simulink model "TC_model"  (R2013a)
settings: Solver=ode45  StartTime=0.0  StopTime=10.0  RelTol=1e-3
undefined symbols (not defined in the file): ctrl_sat, DiscIntNeverNeededParam
libraries: powerlib x7
settings Model: CovModelRefEnable=off  Creator=Copy864  LastModifiedBy=Copy864
settings DataIOCC: LimitDataPoints=off  SaveFormat=StructureWithTime
settings DebuggingCC: UnderspecifiedInitializationDetection=Simplified  MergeDetectMultiDrivingBlocksExec=error  SolverPrmCheckMsg=none  FrameProcessingCompatibilityMsg=error  StateNameClashWarn=none
settings HardwareCC: ProdBitPerPointer=64  ProdLargestAtomicFloat=Float  ProdIntDivRoundTo=Zero  ProdEndianess=LittleEndian  ProdHWDeviceType=Specified
settings ModelReferenceCC: PropagateSignalLabelsOutOfModel=on
settings GRTTargetCC: CodeReplacementLibrary=C89/C90 (ANSI)
settings ConfigurationSet: Description=Simscape Multibody

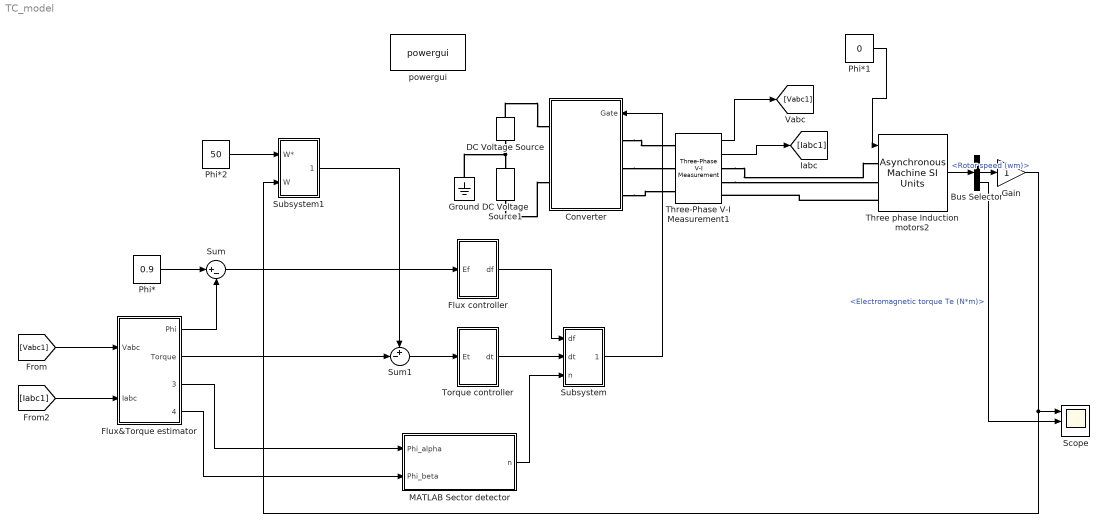
== system TC_model ==
  Bus Selector : BusSelector  OutputSignals=Stator measurements.Stator current is_a (A),Mechanical.Rotor speed (wm),Mechanical.Electromagnetic torque Te (N*m)
  Converter : Subsystem
  DC Voltage Source : powerlib/Electrical Sources/DC Voltage Source  Amplitude=250  Measurements=None
  DC Voltage Source1 : powerlib/Electrical Sources/DC Voltage Source  Amplitude=250  Measurements=None
  Flux controller : Subsystem
  Flux&Torque estimator : Subsystem
  Gain : Gain
  Ground : powerlib/Elements/Ground  LConnTagsString=a
  MATLAB Sector detector : MATLAB Function  TreatAsAtomicUnit=on
      settings: PermitHierarchicalResolution=ParametersOnly
  Phi* : Constant  Value=0.9
  Phi*1 : Constant  Value=0
  Phi*2 : Constant  Value=50
  Scope : Scope  NumInputPorts=3
      settings: TimeRange=auto  MaxDataPoints=5000  SaveName=ScopeData  YMin=-16.0259~-157.28143~-1.00000  YMax=144.23311~146.13243~1.00000  SampleTime=-1
  Subsystem : Subsystem
  Subsystem1 : Subsystem
  Sum : Sum  Inputs=|+-
  Sum1 : Sum  Inputs=+-|
  Three phase Induction motors2 : powerlib/Machines/Asynchronous Machine SI Units  RotorType=Squirrel-cage  PresetModel=No  MechanicalLoad=Torque Tm  ShowDetailedParameters=on  ReferenceFrame=Rotor  Units=SI  MeasurementBus=off  NominalParameters=[500000 460 60]  Stator=[0.6837 0.004152]  Rotor=[0.451 0.004152]  Cage1=[0.4155 0.002066]  Cage2=[0.4168 0.0003495]  Lm=0.1486  Mechanical=[0.05 0.02791 1]  PolePairs=2  InitialConditions=[1 0 0 0 0 0 0 0]  SimulateSaturation=off  Saturation=[14.03593122, 27.81365428, 53.79336849, 72.68890987, 97.98006896, 148.6815601, 215.7428561, 302.9841135, 428.7778367 ; 230, 322, 414, 460, 506, 552, 598, 644, 690]  LoadFlowParameters=1492000  TsPowergui=0  TsBlock=2*10^-6  IterativeModel=Trapezoidal non iterative  IterativeDiscreteModel=Trapezoidal iterative (alg. loop)  Pmec=1.492e+006
  Three-Phase V-I Measurement1 : powerlib/Measurements/Three-Phase V-I Measurement  VoltageMeasurement=phase-to-ground  SetLabelV=off  LabelV=Vabc  Vpu=off  VpuLL=off  CurrentMeasurement=yes  SetLabelI=off  LabelI=Iabc  Ipu=off  Pbase=100e6  Vbase=500e3  OutputType=Complex  PhasorSimulation=off  PSBequivalent=0
  "Torque controller " : Subsystem
  powergui : powerlib/powergui  Priority=1  SimulationMode=Discrete  SolverType=Backward Euler  SampleTime=2e-6  frequency=60  SPID=on  DisableSnubberDevices=off  DisableRonSwitches=off  DisableVfSwitches=off  SwTol=0  DisplayEquations=off  Interpol=off  ExternalGateDelay=off  methode=off  Ts=100  FunctionMessages=off  echomessages=off  HookPort=off  EnableUseOfTLC=off  x0status=blocks  frequencyindice=0  Pbase=100e6  ErrMax=1e-4  Iterations=50  UnitsV=kV  UnitsW=MW  buscounter=0  RestoreLinks=warning  ResistiveCurrentMeasurement=off  Frange=[0:2:500]  Ylog=off  Xlog=on  ShowGrid=off  save=off  variable=ZData  structure=0  ZoomFFT=off  StartTime=0.0  cycles=1  DisplayStyle=1  fundamental=60  FreqAxis=off  MaxFrequency=1000  frequencyindicesteady=1  RmsSteady=1  display=off
  wires:
  Three-Phase V-I Measurement1/2 -> [Iabc1]
  [Vabc1] -> Flux&Torque estimator/1(Vabc)
  [Iabc1] -> Flux&Torque estimator/2(Iabc)
  Flux&Torque estimator/3(Phi_alpha) -> MATLAB Sector detector/1(Phi_alpha)
  Flux&Torque estimator/4(Phi_beta) -> MATLAB Sector detector/2(Phi_beta)
  Flux&Torque estimator/2(Torque) -> Sum1/2
  Flux&Torque estimator/1(Phi) -> Sum/2
  Phi*/1 -> Sum/1
  Sum/1 -> Flux controller/1(Ef)
  Sum1/1 -> "Torque controller "/1(Et)
  Flux controller/1(df) -> Subsystem/1(df)
  "Torque controller "/1(dt) -> Subsystem/2(dt)
  MATLAB Sector detector/1(n) -> Subsystem/3(n)
  Subsystem/1(Gate) -> Converter/1("Gate ")
  Three phase Induction motors2/1 -> Bus Selector/1
  Bus Selector/2 -> Gain/1  "<Rotor speed (wm)>"
  Phi*2/1 -> Subsystem1/1(W*)
  Gain/1 -> Subsystem1/2(W), Scope/1
  Bus Selector/3 -> Scope/2  "<Electromagnetic torque Te (N*m)>"
  Three-Phase V-I Measurement1/1 -> [Vabc1]
  Phi*1/1 -> Three phase Induction motors2/1
  Subsystem1/1(Te*) -> Sum1/1
  connections:
  Three phase Induction motors2/LConn3 -- Three-Phase V-I Measurement1/RConn3
  Converter/LConn2 -- Three-Phase V-I Measurement1/LConn2
  Converter/LConn1 -- Three-Phase V-I Measurement1/LConn1
  Three-Phase V-I Measurement1/RConn1 -- Three phase Induction motors2/LConn1
  Converter/LConn3 -- Three-Phase V-I Measurement1/LConn3
  Three-Phase V-I Measurement1/RConn2 -- Three phase Induction motors2/LConn2
  DC Voltage Source/RConn1 -- Converter/RConn1
  DC Voltage Source/LConn1 -- Ground/LConn1 -- DC Voltage Source1/RConn1
  DC Voltage Source1/LConn1 -- Converter/RConn2

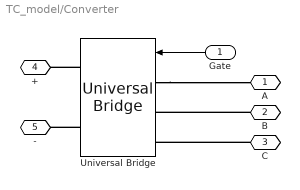
== system TC_model/Converter ==
  "Gate " : Inport
  Universal Bridge : powerlib/Power Electronics/Universal Bridge  Arms=3  SnubberResistance=1e5  SnubberCapacitance=inf  Device=IGBT / Diodes  Ron=1e-3  Lon=0  ForwardVoltages="[  0  0  ]"  ForwardVoltage=0  GTOparameters=[ 10e-6 , 20e-6 ]  IGBTparameters=[ 1e-6 , 2e-6 ]  Measurements=None  Measurements_2=None  converterType=Rectifier
  A : PMIOPort  Port=1  Side=Left
  B : PMIOPort  Port=2  Side=Left
  C : PMIOPort  Port=3  Side=Left
  + : PMIOPort  Port=4  Side=Right
  - : PMIOPort  Port=5  Side=Right
  wires:
  "Gate "/1 -> Universal Bridge/1
  connections:
  C/RConn1 -- Universal Bridge/LConn3
  Universal Bridge/RConn1 -- +/RConn1
  Universal Bridge/LConn1 -- A/RConn1
  Universal Bridge/RConn2 -- -/RConn1
  B/RConn1 -- Universal Bridge/LConn2

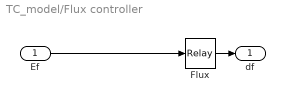
== system TC_model/Flux controller ==
  Ef : Inport
  Flux : Relay  OnSwitchValue=0.005  OffSwitchValue=-0.005
  df : Outport
  wires:
  Ef/1 -> Flux/1
  Flux/1 -> df/1

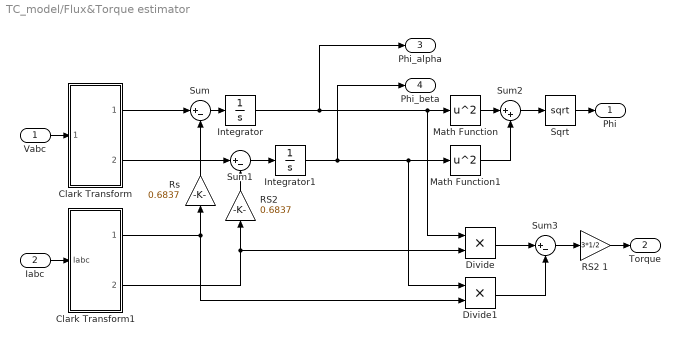
== system TC_model/Flux&Torque estimator ==
  Vabc : Inport
  Iabc : Inport  Port=2
  Clark Transform : Subsystem
  Clark Transform1 : Subsystem
  Divide : Product  Inputs=**
  Divide1 : Product  Inputs=**
  Integrator : Integrator
  Integrator1 : Integrator
  Math Function : Math  Operator=square  SaturateOnIntegerOverflow=on
  Math Function1 : Math  Operator=square  SaturateOnIntegerOverflow=on
  "RS2 " : Gain  Gain=0.6837
  RS2 1 : Gain  Gain=3*1/2
  Rs : Gain  Gain=0.6837
  Sqrt : Sqrt  SaturateOnIntegerOverflow=on
  Sum : Sum  Inputs=|+-
  Sum1 : Sum  Inputs=|+-
  Sum2 : Sum  Inputs=|++
  Sum3 : Sum  Inputs=|+-
  Phi : Outport
  Torque : Outport  Port=2
  Phi_alpha : Outport  Port=3
  Phi_beta : Outport  Port=4
  wires:
  Math Function1/1 -> Sum2/2
  Sum2/1 -> Sqrt/1
  Integrator/1 -> Phi_alpha/1, Divide/1, Math Function/1
  RS2 1/1 -> Torque/1
  Clark Transform1/2("Ibeta ") -> "RS2 "/1, Divide/2
  Rs/1 -> Sum/2
  "RS2 "/1 -> Sum1/2
  Clark Transform1/1(Ialpha) -> Divide1/2, Rs/1
  Divide/1 -> Sum3/1
  Integrator1/1 -> Phi_beta/1, Divide1/1, Math Function1/1
  Sum1/1 -> Integrator1/1
  Math Function/1 -> Sum2/1
  Clark Transform/1(Valpha) -> Sum/1
  Clark Transform/2("Vbeta ") -> Sum1/1
  Divide1/1 -> Sum3/2
  Sum/1 -> Integrator/1
  Sum3/1 -> RS2 1/1
  Vabc/1 -> Clark Transform/1(Vabc)
  Iabc/1 -> Clark Transform1/1(Iabc)
  Sqrt/1 -> Phi/1

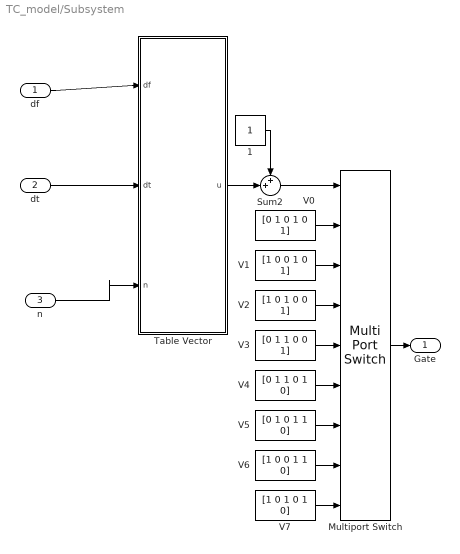
== system TC_model/Subsystem ==
  df : Inport
  dt : Inport  Port=2
  n : Inport  Port=3
  1 : Constant
  Multiport Switch : MultiPortSwitch  Inputs=8
  Sum2 : Sum  Inputs=++|
  Table Vector : MATLAB Function  TreatAsAtomicUnit=on
      settings: PermitHierarchicalResolution=ParametersOnly
  V0 : Constant  Value=[0 1 0 1 0 1]
  V1 : Constant  Value=[1 0 0 1 0 1]
  V2 : Constant  Value=[1 0 1 0 0 1]
  "V3 " : Constant  Value=[0 1 1 0 0 1]
  V4 : Constant  Value=[0 1 1 0 1 0]
  V5 : Constant  Value=[0 1 0 1 1 0]
  V6 : Constant  Value=[1 0 0 1 1 0]
  V7 : Constant  Value=[1 0 1 0 1 0]
  Gate : Outport
  wires:
  "V3 "/1 -> Multiport Switch/5
  V7/1 -> Multiport Switch/9
  V5/1 -> Multiport Switch/7
  1/1 -> Sum2/1
  V2/1 -> Multiport Switch/4
  V1/1 -> Multiport Switch/3
  dt/1 -> Table Vector/2(dt)
  V4/1 -> Multiport Switch/6
  V0/1 -> Multiport Switch/2
  Table Vector/1(u) -> Sum2/2
  Sum2/1 -> Multiport Switch/1
  V6/1 -> Multiport Switch/8
  n/1 -> Table Vector/3(n)
  Multiport Switch/1 -> Gate/1
  df/1 -> Table Vector/1(df)

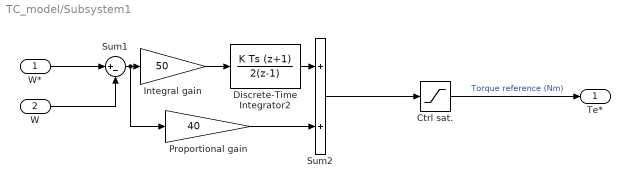
== system TC_model/Subsystem1 ==
  W* : Inport
  W : Inport  Port=2
  Ctrl sat. : Saturate  UpperLimit=1e6  LowerLimit=-2000
  Discrete-Time Integrator2 : DiscreteIntegrator  IntegratorMethod=Integration: Trapezoidal  SampleTime=-1  UpperSaturationLimit=ctrl_sat(2)  LowerSaturationLimit=ctrl_sat(1)  ICPrevOutput=DiscIntNeverNeededParam  ICPrevScaledInput=DiscIntNeverNeededParam
  Integral gain : Gain  Gain=50  SaturateOnIntegerOverflow=on  OutDataTypeStr=Inherit: Same as input  ParamDataTypeStr=Inherit: Same as input
  Proportional gain : Gain  Gain=40  SaturateOnIntegerOverflow=on  OutDataTypeStr=Inherit: Same as input  ParamDataTypeStr=Inherit: Same as input
  Sum1 : Sum  Inputs=|+-  SaturateOnIntegerOverflow=on  InputSameDT=on  OutDataTypeStr=Inherit: Same as first input
  Sum2 : Sum  SaturateOnIntegerOverflow=on  InputSameDT=on  OutDataTypeStr=Inherit: Same as first input
  Te* : Outport
  wires:
  Sum2/1 -> Ctrl sat./1
  Integral gain/1 -> Discrete-Time Integrator2/1
  Discrete-Time Integrator2/1 -> Sum2/1
  Sum1/1 -> Integral gain/1, Proportional gain/1
  Proportional gain/1 -> Sum2/2
  W*/1 -> Sum1/1
  W/1 -> Sum1/2
  Ctrl sat./1 -> Te*/1  "Torque reference (Nm)"

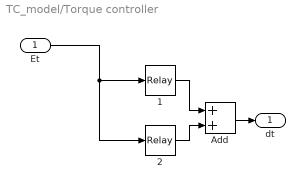
== system TC_model/Torque controller  ==
  Et : Inport
  "1 " : Relay  OnSwitchValue=1  OffSwitchValue=0
  2 : Relay  OnSwitchValue=0  OffSwitchValue=-1  OnOutputValue=0  OffOutputValue=-1
  Add : Sum
  dt : Outport
  wires:
  Et/1 -> "1 "/1, 2/1
  Add/1 -> dt/1
  "1 "/1 -> Add/1
  2/1 -> Add/2

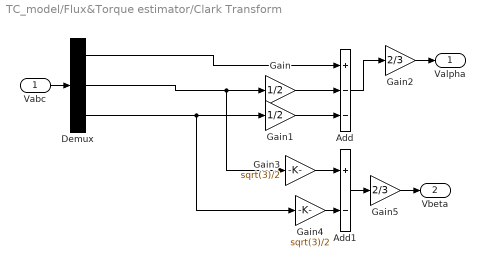
== system TC_model/Flux&Torque estimator/Clark Transform ==
  Vabc : Inport
  Add : Sum  Inputs=+--
  Add1 : Sum  Inputs=+-
  Demux : Demux  Outputs=3
  Gain : Gain  Gain=1/2
  Gain1 : Gain  Gain=1/2
  Gain2 : Gain  Gain=2/3
  Gain3 : Gain  Gain=sqrt(3)/2
  Gain4 : Gain  Gain=sqrt(3)/2
  Gain5 : Gain  Gain=2/3
  Valpha : Outport
  "Vbeta " : Outport  Port=2
  wires:
  Demux/3 -> Gain4/1, Gain1/1
  Gain1/1 -> Add/3
  Gain4/1 -> Add1/2
  Demux/1 -> Add/1
  Demux/2 -> Gain3/1, Gain/1
  Gain3/1 -> Add1/1
  Add/1 -> Gain2/1
  Gain/1 -> Add/2
  Add1/1 -> Gain5/1
  Vabc/1 -> Demux/1
  Gain2/1 -> Valpha/1
  Gain5/1 -> "Vbeta "/1

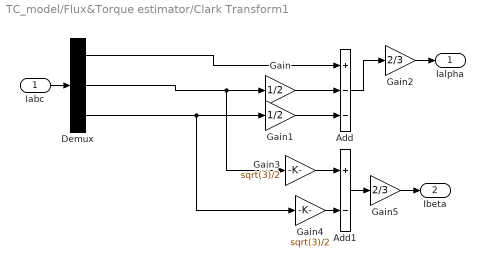
== system TC_model/Flux&Torque estimator/Clark Transform1 ==
  Iabc : Inport
  Add : Sum  Inputs=+--
  Add1 : Sum  Inputs=+-
  Demux : Demux  Outputs=3
  Gain : Gain  Gain=1/2
  Gain1 : Gain  Gain=1/2
  Gain2 : Gain  Gain=2/3
  Gain3 : Gain  Gain=sqrt(3)/2
  Gain4 : Gain  Gain=sqrt(3)/2
  Gain5 : Gain  Gain=2/3
  Ialpha : Outport
  "Ibeta " : Outport  Port=2
  wires:
  Gain5/1 -> "Ibeta "/1
  Gain2/1 -> Ialpha/1
  Iabc/1 -> Demux/1
  Add1/1 -> Gain5/1
  Gain/1 -> Add/2
  Add/1 -> Gain2/1
  Gain3/1 -> Add1/1
  Demux/2 -> Gain/1, Gain3/1
  Demux/1 -> Add/1
  Gain4/1 -> Add1/2
  Gain1/1 -> Add/3
  Demux/3 -> Gain1/1, Gain4/1

== matlab function TC_model/Subsystem/Table Vector ==
  data: df input; u output; dt input; n input
function u = fcn(df, dt , n)
u = 0;
if (df == 1) & (dt == 1) & (n == 1)
    u =2;   
end

if (df == 1) & (dt == 0) & (n == 1)
    u =7;   
end

if (df == 1) & (dt == -1) & (n == 1)
    u =6;   
end
%%%%%%%%%%%%%%%%%%%%%%%%%%%%%%%
if (df == 1) & (dt == 1) & (n == 2)
    u =3;   
end
if (df == 1) & (dt == 0) & (n == 2)
    u =0;   
end
if (df == 1) & (dt == -1) & (n == 2)
    u =1;   
end
%%%%%%%%%%%%%%%%%%%%%%%%%%%%%
if (df == 1) & (dt == 1) & (n == 3)
    u =4;   
end
if (df == 1) & (dt == 0) & (n == 3)
    u =7;   
end
if (df == 1) & (dt == -1) & (n == 3)
    u =2;   
end
%%%%%%%%%%%%%%%%%%%%%%%%%%%%%
if (df == 1) & (dt == 1) & (n == 4)
    u =5;   
end
if (df == 1) & (dt == 0) & (n == 4)
    u =0;   
end
if (df == 1) & (dt == -1) & (n == 4)
    u =3;   
end
%%%%%%%%%%%%%%%%%%%%%%%%%%%%%
if (df == 1) & (dt == 1) & (n == 5)
    u =6;   
end
if (df == 1) & (dt == 0) & (n == 5)
    u =7;   
end
if (df == 1) & (dt == -1) & (n == 5)
    u =4;   
end
%%%%%%%%%%%%%%%%%%%%%%%%%%%%%
if (df == 1) & (dt == 1) & (n == 6)
    u =1;   
end
if (df == 1) & (dt == 0) & (n == 6)
    u =0;   
end
if (df == 1) & (dt == -1) & (n == 6)
    u =5;   
end

%%%%%%%%%%%%%%%%%%%%%%%%%%%
%%%%%%%%%%%%%%%%%%%%%%%%%%%%%%%%%%%%%%%%%%%%%%

if (df == 0) & (dt == 1) & (n == 1)
    u =3;   
end

if (df == 0) & (dt == 0) & (n == 1)
    u =0;   
end

if (df == 0) & (dt == -1) & (n == 1)
    u =5;   
end
%%%%%%%%%%%%%%%%%%%%%%%%%%%%%%%
if (df == 0) & (dt == 1) & (n == 2)
    u =4;   
end
if (df == 0) & (dt == 0) & (n == 2)
    u =7;   
end
if (df == 0) & (dt == -1) & (n == 2)
    u =6;   
end
%%%%%%%%%%%%%%%%%%%%%%%%%%%%%
if (df == 0) & (dt == 1) & (n == 3)
    u =5;   
end
if (df == 0) & (dt == 0) & (n == 3)
    u =0;   
end
if (df == 0) & (dt == -1) & (n == 3)
    u =1;   
end
%%%%%%%%%%%%%%%%%%%%%%%%%%%%%
if (df == 0) & (dt == 1) & (n == 4)
    u =6;   
end
if (df == 0) & (dt == 0) & (n == 4)
    u =7;   
end
if (df == 0) & (dt == -1) & (n == 4)
    u =2;   
end
%%%%%%%%%%%%%%%%%%%%%%%%%%%%%
if (df == 0) & (dt == 1) & (n == 5)
    u =1;   
end
if (df == 0) & (dt == 0) & (n == 5)
    u =0;   
end
if (df == 0) & (dt == -1) & (n == 5)
    u =3;   
end
%%%%%%%%%%%%%%%%%%%%%%%%%%%%%
if (df == 0) & (dt == 1) & (n == 6)
    u =2;   
end
if (df == 0) & (dt == 0) & (n == 6)
    u =7;   
end
if (df == 0) & (dt == -1) & (n == 6)
    u =4;   
end

== matlab function TC_model/MATLAB Sector detector ==
  data: Phi_alpha input; n output; Phi_beta input
function n = Selector(Phi_alpha,Phi_beta)
n = 0;
deta = atan2(Phi_beta,Phi_alpha);

if (deta>= -pi/6) & (deta<pi/6)
    n = 1;
end

if (deta>= pi/6) & (deta<pi/2)
    n = 2;
end

if (deta>= pi/2) & (deta< 5*pi/6)
    n = 3;
end

if (deta>=5*pi/6) & (deta< pi)
    n = 4;
end
if (deta>=-pi) & (deta< -5*pi/6)
    n = 4;
end
if (deta>=-5*pi/6) & (deta< -1*pi/2)
    n = 5;
end

if (deta>= -1*pi/2) & (deta< -1*pi/6)
    n = 6;
end
